simulink model "chap5_1sim"  (Simulink 6.3)
settings: Solver=ode45  StartTime=0.0  StopTime=100  FixedStep=0.001  RelTol=1e-3
settings Model: LastModifiedBy=Administrator  ExtModeTrigMode=oneshot  ExtModeArmWhenConnect=off  StrictBusMsg=None
settings DataIOCC: LimitDataPoints=off  SignalLoggingName=sigsOut
settings OptimizationCC: BooleanDataType=off
settings DebuggingCC: SolverPrmCheckMsg=none
settings HardwareCC: TargetUnknown=on

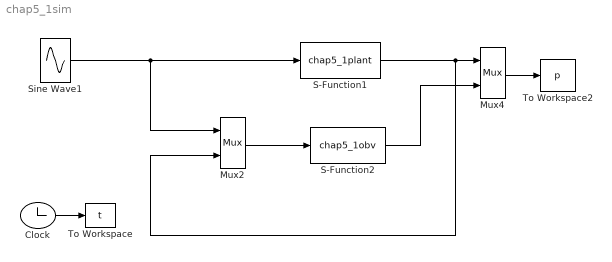
== system chap5_1sim ==
  Clock : Clock
  Mux2 : Mux  Inputs=2
  Mux4 : Mux  Inputs=2
  S-Function1 : S-Function  FunctionName=chap5_1plant
  S-Function2 : S-Function  FunctionName=chap5_1obv
  Sine Wave1 : Sin  Frequency=100  SampleTime=0
  To Workspace : ToWorkspace  VariableName=t  SampleTime=-1  SaveFormat=Array
  To Workspace2 : ToWorkspace  VariableName=p  SampleTime=-1  SaveFormat=Array
  wires:
  S-Function1/1 -> Mux2/2, Mux4/1
  Clock/1 -> To Workspace/1
  Mux4/1 -> To Workspace2/1
  Sine Wave1/1 -> Mux2/1, S-Function1/1
  S-Function2/1 -> Mux4/2
  Mux2/1 -> S-Function2/1
